simulink model "A3_Assignment"  (R2022a)
settings: Solver=FixedStepAuto  StartTime=0.0  StopTime=inf  FixedStep=0.1  RelTol=1e-3
model workspace (MAT data in the model file):
  SL_ROS_VariableLengthArrays_MaxSizes.CommonInfo.ArrayTruncateAction = 'EmitWarning'
  SL_ROS_VariableLengthArrays_MaxSizes.MsgTypeMap = containers.Map
  SL_ROS_VariableLengthArrays_MaxSizes.MsgTypeMap.serialization.keys = {'sensor_msgs/Image'}
  SL_ROS_VariableLengthArrays_MaxSizes.MsgTypeMap.serialization.values{1}(1).PropertyName = 'Data'
  SL_ROS_VariableLengthArrays_MaxSizes.MsgTypeMap.serialization.values{1}(1).DataType = 'uint8'
  SL_ROS_VariableLengthArrays_MaxSizes.MsgTypeMap.serialization.values{1}(1).MaxLength = 921600
  SL_ROS_VariableLengthArrays_MaxSizes.MsgTypeMap.serialization.values{1}(2).PropertyName = 'Encoding'
  SL_ROS_VariableLengthArrays_MaxSizes.MsgTypeMap.serialization.values{1}(2).DataType = 'uint8'
  SL_ROS_VariableLengthArrays_MaxSizes.MsgTypeMap.serialization.values{1}(2).MaxLength = 128
  SL_ROS_VariableLengthArrays_MaxSizes.MsgTypeMap.serialization.uniformity = 0
  SL_ROS_VariableLengthArrays_MaxSizes.MsgTypeMap.serialization.keyType = 'char'
  SL_ROS_VariableLengthArrays_MaxSizes.MsgTypeMap.serialization.valueType = 'any'
undefined symbols (not defined in the file or in its folder): Angular, gray, Linear, Rec, SDTV
libraries: robotlib x6, simulink x2, visionstatistics x1, visionconversions x1, visiontextngfix x1
settings Model: Creator=jacopo  LastModifiedBy=Jacopo
settings OptimizationCC: EnhancedBackFolding=on  PassReuseOutputArgsAs=Individual arguments  ZeroExternalMemoryAtStartup=off  ZeroInternalMemoryAtStartup=off  MaxStackSize=64  OptimizeBlockOrder=speed  DifferentSizesBufferReuse=on  OptimizationCustomize=off  EfficientTunableParamExpr=on
settings DebuggingCC: ParameterTunabilityLossMsg=error
settings HardwareCC: ProdBitPerPointer=32  ProdBitPerSizeT=32  ProdBitPerPtrDiffT=32  ProdLargestAtomicFloat=None  ProdIntDivRoundTo=Undefined  ProdEndianess=Unspecified  ProdWordSize=32  ProdHWDeviceType=Generic->Unspecified (assume 32-bit Generic)
settings SFSimCC: MATLABDynamicMemAlloc=off
settings RTWCC: SystemTargetFile=ert.tlc  HardwareBoard=Robot Operating System (ROS)  TLCOptions="-aInlineSetEventsForThisBaseRateFcn=TLC_FALSE -aSuppressMultiTaskScheduler=TLC_FALSE  -aRateBasedStepFcn=0"  TemplateMakefile=ert_default_tmf  Toolchain=Catkin  TargetLang=C++
settings CodeAppCC: ForceParamTrailComments=on  IgnoreCustomStorageClasses=off  OperatorAnnotations=on  SimulinkDataObjDesc=on  SFDataObjDesc=on  InsertBlockDesc=on

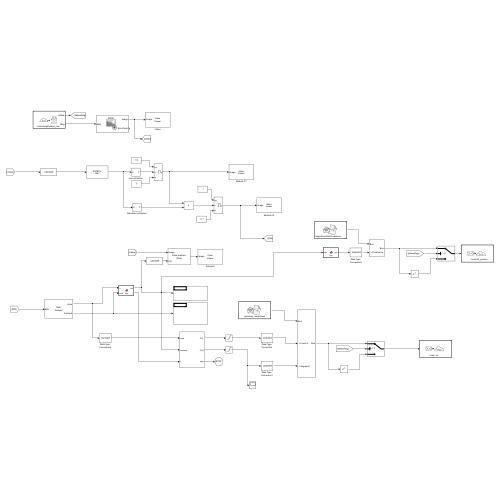
[thumbnail: Simulink's stored preview of the top-level diagram]
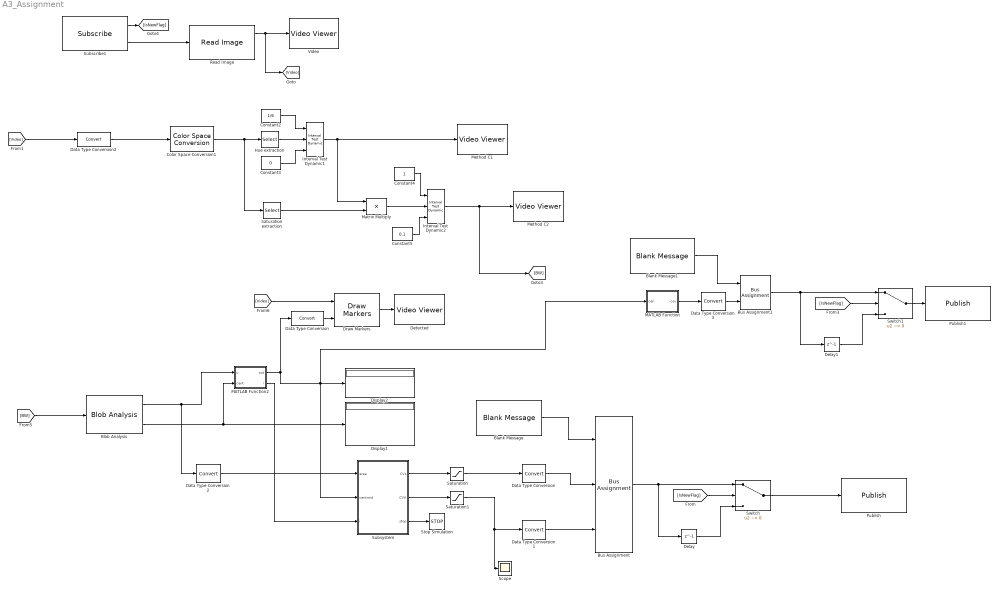
== system A3_Assignment ==
  Blank Message : robotlib/Blank Message  messageClass=Message  entityType=geometry_msgs/Twist  messageType=geometry_msgs/Twist  SampleTime=inf  legacyBusStruct=off
  Blank Message1 : robotlib/Blank Message  messageClass=Message  entityType=geometry_msgs/PoseWithCovariance  messageType=geometry_msgs/PoseWithCovariance  SampleTime=inf  legacyBusStruct=off
  Blob Analysis : visionstatistics/Blob Analysis  Tag=vipblks_row_conv  area=on  centroid=on  bBox=off  majorAxis=off  minorAxis=off  angle=off  eccentricity=off  equivDiameterSq=off  extent=off  perimeter=off  outDT=double  conn=8  isLabel=off  maxBlobs=2  warnIfNumBlobsExceeded=on  isCount=off  useMinArea=off  minArea=0  useMaxArea=off  maxArea=intmax('uint32')  excludeBorderBlob=off  isOutVarDim=off  isFill=on  fillValues=-1  roundingMode=Floor  overflowMode=off  prodOutputMode=Binary point scaling  prodOutputWordLength=32  prodOutputFracLength=16  accumMode=Binary point scaling  accumWordLength=32  accumFracLength=0  outputMode=Binary point scaling  outputWordLength=32  outputFracLength=16  firstCoeffMode=Binary point scaling  firstCoeffWordLength=16  firstCoeffFracLength=14  secondCoeffMode=Binary point scaling  secondCoeffWordLength=32  secondCoeffFracLength=16
  Bus Assignment : BusAssignment  AssignedSignals=Linear.X,Angular.Z
  Bus Assignment1 : BusAssignment  AssignedSignals=Covariance
  Color Space Conversion1 : visionconversions/Color Space  Conversion  conversion=Obsolete  conversionActive=R'G'B' to HSV  wp_str=D65  rec=Rec. 601 (SDTV)  sys=1125/60/2:1  imagePorts=One multidimensional signal
  Constant2 : Constant  Value=1/6
  Constant3 : Constant  Value=0
  Constant4 : Constant
  Constant5 : Constant  Value=0.1
  Data Type Conversion{,,1..2,2..3} (6 alike) : DataTypeConversion  SaturateOnIntegerOverflow=off  RndMeth=Floor
  Delay : Delay  DelayLength=1
  Delay1 : Delay  DelayLength=1
  Detected : VideoViewer  colormapValue=gray(256)  FigPos=[98 798 583 363]
  Display1 : Display
  Display2 : Display
  Draw Markers : visiontextngfix/Draw Markers  shape=Plus  size=30  fill=off  fillClrSource=Specify via dialog  display=User-specified value  intensity=200  color=[255 0 0]  opacity=0.6  viewport=Entire image  antialiasing=off  inType=Obsolete  imagePorts=One multidimensional signal  roundingMode=Floor  overflowMode=off  memoryMode=Specify word length  memoryWordLength=16  memoryFracLength=15  prodOutputMode=Binary point scaling  prodOutputWordLength=32  prodOutputFracLength=14
  Hue extraction : Selector  NumberOfDimensions=3  InputPortWidth=3  IndexOptions=Index vector (dialog),Index vector (dialog),Index vector (dialog)  Indices=[1:480],[1:640],1  OutputSizes=1,1,1
  Interval Test Dynamic1 : simulink/Logic and Bit Operations/Interval Test Dynamic  IntervalClosedRight=on  IntervalClosedLeft=on  OutDataTypeStr=boolean
  Interval Test Dynamic2 : simulink/Logic and Bit Operations/Interval Test Dynamic  IntervalClosedRight=on  IntervalClosedLeft=on  OutDataTypeStr=boolean
  MATLAB Function : MATLAB Function  TreatAsAtomicUnit=on
  MATLAB Function2 : MATLAB Function  TreatAsAtomicUnit=on
  Matrix Multiply : Product
  Method C1 : VideoViewer  colormapValue=gray(256)  FigPos=[314 762 591 337]
  Method C2 : VideoViewer  colormapValue=gray(256)  FigPos=[870 589 571 351]
  Publish : robotlib/Publish  topicSource=Select from ROS network  topic=/cmd_vel  messageType=geometry_msgs/Twist  legacyBusStruct=off  messageQueueLength=1
  Publish1 : robotlib/Publish  topicSource=Specify your own  topic=/centroid_position  messageType=geometry_msgs/PoseWithCovariance  legacyBusStruct=off  messageQueueLength=1
  Read Image : robotlib/Read Image  MaximumImageSize=[480, 640]  ImageEncoding=rgb8  ShowAlphaOutput=off  ShowErrorCodeOutput=on  VariableSizeOutputs=off
  Saturation : Saturate  UpperLimit=0.2  LowerLimit=-0.2
  Saturation extraction : Selector  NumberOfDimensions=3  InputPortWidth=3  IndexOptions=Index vector (dialog),Index vector (dialog),Index vector (dialog)  Indices=[1:480],[1:640],2  OutputSizes=1,1,1
  Saturation1 : Saturate  UpperLimit=0.4  LowerLimit=-0.4
  Scope : Scope
  Stop Simulation : Stop
  Subscribe1 : robotlib/Subscribe  topicSource=Select from ROS network  topic=/camera/rgb/image_raw  messageType=sensor_msgs/Image  SampleTime=-1  legacyBusStruct=off  messageQueueLength=1
  Subsystem : Subsystem
  Switch : Switch  Criteria=u2 ~= 0  SaturateOnIntegerOverflow=off  InputSameDT=off
  Switch1 : Switch  Criteria=u2 ~= 0  SaturateOnIntegerOverflow=off  InputSameDT=off
  Video : VideoViewer  colormapValue=gray(256)  FigPos=[660 793 576 345]
  wires:
  Subscribe1/2 -> Read Image/1
  Read Image/1 -> [Video], Video/1
  Draw Markers/1 -> Detected/1
  [BW] -> Blob Analysis/1
  MATLAB Function2/1(out) -> Data Type Conversion/1, MATLAB Function/1(cen), Subsystem/2(centroid), Display2/1
  [Video] -> Draw Markers/1
  Blob Analysis/2 -> MATLAB Function2/2(cent), Display1/1
  Data Type Conversion/1 -> Draw Markers/2
  Blob Analysis/1 -> MATLAB Function2/1(u), Data Type Conversion2/1
  Constant3/1 -> Interval Test Dynamic1/3
  Data Type Conversion2/1 -> Color Space Conversion1/1
  Hue extraction/1 -> Interval Test Dynamic1/2
  Constant2/1 -> Interval Test Dynamic1/1
  [Video] -> Data Type Conversion2/1
  Interval Test Dynamic1/1 -> Matrix Multiply/1, Method C1/1
  Color Space Conversion1/1 -> Saturation extraction/1, Hue extraction/1
  Saturation extraction/1 -> Matrix Multiply/2
  Interval Test Dynamic2/1 -> [BW], Method C2/1
  Matrix Multiply/1 -> Interval Test Dynamic2/2
  Constant4/1 -> Interval Test Dynamic2/1
  Constant5/1 -> Interval Test Dynamic2/3
  Blank Message/1 -> Bus Assignment/1
  Data Type Conversion/1 -> Bus Assignment/2
  Data Type Conversion1/1 -> Bus Assignment/3
  Subscribe1/1 -> [IsNewFlag]
  Saturation/1 -> Data Type Conversion/1
  Saturation1/1 -> Data Type Conversion1/1, Scope/1
  Delay/1 -> Switch/3
  [IsNewFlag] -> Switch/2
  Bus Assignment/1 -> Delay/1, Switch/1
  Switch/1 -> Publish/1
  Data Type Conversion2/1 -> Subsystem/1(area)
  MATLAB Function2/2(i) -> Subsystem/3(i)
  Subsystem/1(CVL) -> Saturation/1
  Subsystem/2(CVA) -> Saturation1/1
  Subsystem/3(stop) -> Stop Simulation/1
  Blank Message1/1 -> Bus Assignment1/1
  MATLAB Function/1(cov) -> Data Type Conversion3/1
  Data Type Conversion3/1 -> Bus Assignment1/2
  Delay1/1 -> Switch1/3
  [IsNewFlag] -> Switch1/2
  Bus Assignment1/1 -> Delay1/1, Switch1/1
  Switch1/1 -> Publish1/1

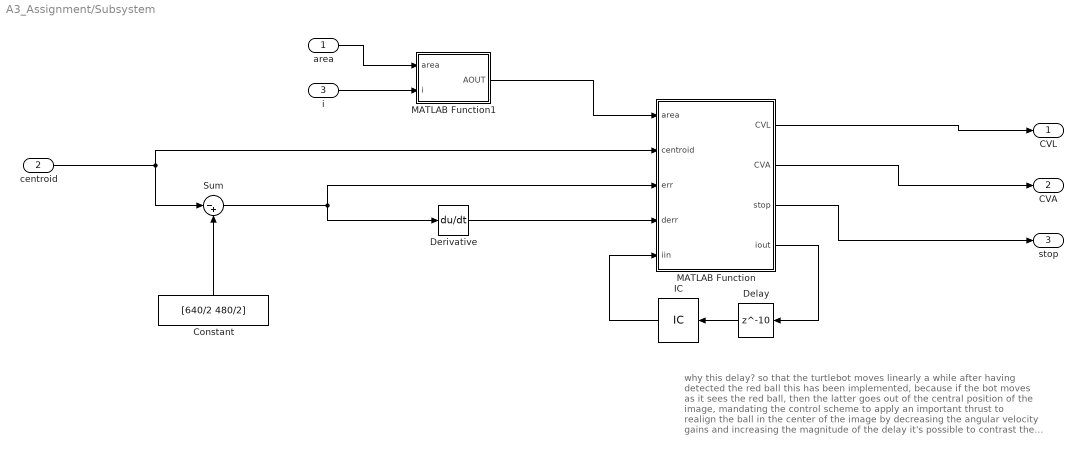
== system A3_Assignment/Subsystem ==
  note: why this delay? so that the turtlebot moves linearly a while after
      | having detected the red ball
      | this has been implemented, because if the bot moves as it sees
      | the red ball, then the latter goes out of the central position of the image,
      | mandating the control scheme to apply an important thrust to realign
      | the ball in the center of the image
      | by decreasing the angular velocity gains and increasing the magnitude
      | of the delay it's possible to contrast the wobbly motion, caused by
      | a synergic cooperation of high gains and moving linearly too early
  area : Inport
  centroid : Inport  Port=2
  i : Inport  Port=3
  Constant : Constant  Value=[640/2 480/2]  VectorParams1D=off
  Delay : Delay  DelayLength=10
  Derivative : Derivative
  IC : InitialCondition  Value=0
  MATLAB Function : MATLAB Function  TreatAsAtomicUnit=on
  MATLAB Function1 : MATLAB Function  TreatAsAtomicUnit=on
  Sum : Sum  Inputs=|-+
  CVL : Outport
  CVA : Outport  Port=2
  stop : Outport  Port=3
  wires:
  MATLAB Function/3(stop) -> stop/1
  area/1 -> MATLAB Function1/1(area)
  MATLAB Function/2(CVA) -> CVA/1
  MATLAB Function/1(CVL) -> CVL/1
  MATLAB Function1/1(AOUT) -> MATLAB Function/1(area)
  i/1 -> MATLAB Function1/2(i)
  centroid/1 -> Sum/1, MATLAB Function/2(centroid)
  Constant/1 -> Sum/2
  Sum/1 -> Derivative/1, MATLAB Function/3(err)
  Derivative/1 -> MATLAB Function/4(derr)
  Delay/1 -> IC/1
  MATLAB Function/4(iout) -> Delay/1
  IC/1 -> MATLAB Function/5(iin)

== matlab function A3_Assignment/Subsystem/MATLAB Function ==
  data: area input; CVL output; centroid input; CVA output; err input; stop output; derr input; iin input; iout output
function [CVL, CVA, stop, iout] = fcn(area, centroid, err, derr, iin)

NC = 2; % max number of centroids
NoCV = - ones(NC, 2);

if centroid == NoCV
    CVL = 0;
    CVA = 0.2;
    iout = 0;
else
    iout = 1;
    kPL = 0.05;
    kPA = 0.003;
    kDA = 0.01*0;
    kIA = 0;
    
    ERR = err(1);
    dERR = derr(1);

    if iin == 1
        CVL = kPL*area;
    else
        CVL = 0;
    end

    CVA = kPA*ERR + kDA*dERR + kIA*intERR;
end

maxA = 0.9*(640*480);

if area < maxA
    stop = 0;
else
    CVL = 0;
    CVA = 0;
    stop = 1;
end

== matlab function A3_Assignment/MATLAB Function2 ==
  data: u input; cent input; out output; i output
function [out, i]  = fcn(u,cent)

[~,i] = max(u);

if ~isempty(i)
    out = cent(i,:);
else 
    out = [0,0];
end

== matlab function A3_Assignment/Subsystem/MATLAB Function1 ==
  data: area input; AOUT output; i input
function AOUT = fcn(area, i)

AOUT = area(i, 1);

== matlab function A3_Assignment/MATLAB Function ==
  data: cen input; cov output
function cov = fcn(cen)

cov = [cen zeros(1, 34)];
